simulink model "arbeitspunkt"  (Simulink 7.0)
settings: Solver=FixedStepDiscrete  SolverMode=SingleTasking  StartTime=0.0  StopTime=10  FixedStep=0.001  RelTol=1e-3
undefined symbols (not defined in the file or in its folder): National_Instruments, PCI
libraries: rtwinlib x2
settings Model: Creator=Admin  LastModifiedBy=Student  SimulationMode=external  ExtModeTrigDuration=1000000
settings OptimizationCC: InlineInvariantSignals=on
settings DebuggingCC: SaveWithParameterizedLinksMsg=none  SignalResolutionControl=TryResolveAllWithWarning  MultiTaskDSMMsg=warning  MultiTaskCondExecSysMsg=none  StrictBusMsg=None
settings RTWCC: SystemTargetFile=rtwin.tlc  TemplateMakefile=rtwin.tmf  Description=Real-Time Windows Target  ProcessScript=rtwin_make_rtw_hook  IncludeERTFirstTime=on
settings RTWinTargetCC: TargetFcnLib=ansi_tfl_tmw.mat  GenFloatMathFcnCalls=ANSI_C  ModelReferenceCompliant=off  CompOptLevelCompliant=off  PortableWordSizes=off  CCOptimize=on  RebuildAll=on  ExtModeStaticAlloc=on

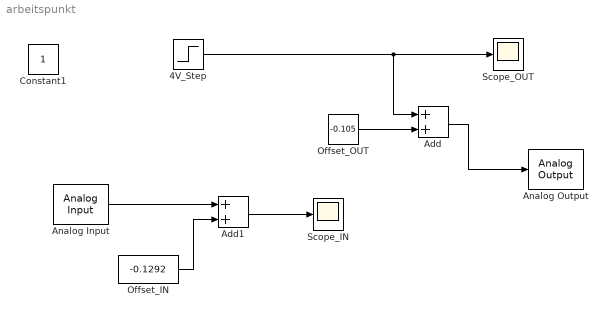
== system arbeitspunkt ==
  4V_Step : Step  After=4  SampleTime=0
  Add : Sum  OutDataType=sfix(16)  OutScaling=2^-10
  Add1 : Sum  OutDataType=sfix(16)  OutScaling=2^-10
  Analog Input : rtwinlib/Analog Input  SampleTime=0.001  DrvName=National_Instruments/PCI-6025E  DrvAddress=4294967295  DrvOptions=[0 1 0 0 0 0]  Channels=1  RangeMode=1  VoltRange=1  DataType=1
      settings: AttributesFormatString=National Instruments\nPCI-6025E [auto]
  Analog Output : rtwinlib/Analog Output  SampleTime=0.001  DrvName=National_Instruments/PCI-6025E  DrvAddress=4294967295  DrvOptions=[0 1 0 0 0 0]  Channels=1  RangeMode=1  VoltRange=1  InitialValue=0  FinalValue=0
      settings: AttributesFormatString=National Instruments\nPCI-6025E [auto]
  Offset_IN : Constant  Value=-0.1292  OutDataType=sfix(16)  OutScaling=2^0
  Offset_OUT : Constant  Value=-0.105  OutDataType=sfix(16)  OutScaling=2^0
  Scope_IN : Scope
      settings: TimeRange=1  YMin=3.5  YMax=4.5  SaveName=ScopeIn_stor  DataFormat=Array
  Scope_OUT : Scope
      settings: TimeRange=1  YMin=2.5  YMax=3.5  SaveName=ScopeOut  DataFormat=Array
  Constant1 : Constant  IOType=siggen  OutDataType=sfix(16)  OutScaling=2^0
  wires:
  Analog Input/1 -> Add1/1
  4V_Step/1 -> Add/1, Scope_OUT/1
  Offset_OUT/1 -> Add/2
  Offset_IN/1 -> Add1/2
  Add/1 -> Analog Output/1
  Add1/1 -> Scope_IN/1
